simulink model "Mathematica_model"  (R2014a)
settings: Solver=ode5  SolverMode=SingleTasking  StartTime=0.0  StopTime=240  FixedStep=1e-6  RelTol=1e-3
InitFcn:
  | Mathematica_model_
values from neighbouring files (symbols this model uses):
  alpha = [alfa 0]    [Mathematica_model_.m]
  Cf = 1000e-6    (= 0.001)    [Mathematica_model_.m]
  CT1 = [34.2 88.9 129.8 148.6 139.3 123.3 69.9 25.5 15.1 10.5]    [Mathematica_model_.m]
  CT2 = [754.4 643.3 977.4 708.0 1119.7 970.2 733.8 708.0 359.8 170.7]    [Mathematica_model_.m]
  distance = [0 1 2 3 4 5 6 7 8 9 10 11 ... (2132 elements, 1x2132)]    [Track_data.mat]
  h_Mem = 5    [Mathematica_model_.m]
  h_Psi_s = 0.01    [Mathematica_model_.m]
  J = 0.043    [Mathematica_model_.m]
  Ki = Kp/Ti    (= 2.8)    [Mathematica_model_.m]
  Kp = 7    [Mathematica_model_.m]
  Kt = Ki/2    (= 1.4)    [Mathematica_model_.m]
  Lf = 1e-6    (= 1e-06)    [Mathematica_model_.m]
  Lm = 249.304e-3    (= 0.249304)    [Mathematica_model_.m]
  Lr = Lm+Llr    (= 0.255875)    [Mathematica_model_.m]
  Ls = Lm+Lls    (= 0.257335)    [Mathematica_model_.m]
  MInv = inv(M)    [Mathematica_model_.m]
  n_paralel = 10    [Mathematica_model_.m]
  n_serial = 162    [Mathematica_model_.m]
  pp = 2    [Mathematica_model_.m]
  Psi_rd_0 = Psi_dq_0(3)    [Mathematica_model_.m]
  Psi_sd_0 = Psi_dq_0(1)    [Mathematica_model_.m]
  Psi_sq_0 = Psi_dq_0(2)    [Mathematica_model_.m]
  Q0 = 4.8*3600    (= 17280)    [Mathematica_model_.m]
  R0 = [73 65 74 83 68 65 65 61 76 87].*1e-4    [Mathematica_model_.m]
  reduction = 2    [Mathematica_model_.m]
  Rf = 2000    [Mathematica_model_.m]
  Rs = 0.847    [Mathematica_model_.m]
  RT1 = [9.76 15 11 5.83 11 11 16 44 53 102].*1e-4    [Mathematica_model_.m]
  RT2 = [24 20 16 22 13 16 22 22 47 153].*1e-4    [Mathematica_model_.m]
  sigma = 1-Lm^2/(Lr*Ls)    (= 0.0560874089476)    [Mathematica_model_.m]
  SoC = [1 0.884 0.769 0.653 0.537 0.421 0.306 0.190 0.074 0]    [Mathematica_model_.m]
  speed = speedOptim    [Mathematica_model_.m]
  tauR = Lr/Rr    (= 0.384890192539)    [Mathematica_model_.m]
  Ts = 25e-6    (= 2.5e-05)    [Mathematica_model_.m]
  Tss = 500e-6    (= 0.0005)    [Mathematica_model_.m]
  Uoc = [4.19 4.06 3.93 3.86 3.8 3.76 3.72 3.6 3.43 3.05]    [Mathematica_model_.m]
  vehicle =     [Track_data.mat]
undefined symbols (not defined in the file or in its folder): DiscIntNeverNeededParam, Voltage
libraries: simulink x3
settings Model: SimulationMode=accelerator  NumberOfSteps=5  Creator=Jan  LastModifiedBy=Jan
settings DataIOCC: SignalLogging=off  DSMLogging=off
settings OptimizationCC: EfficientMapNaN2IntZero=off
settings DebuggingCC: MergeDetectMultiDrivingBlocksExec=error
settings HardwareCC: TargetLongLongMode=on  TargetIntDivRoundTo=Zero  TargetEndianess=LittleEndian  TargetHWDeviceType=MATLAB Host  ProdEqTarget=off
settings CodeAppCC: MaxIdLength=128
settings GRTTargetCC: CombineOutputUpdateFcns=off  GRTInterface=on

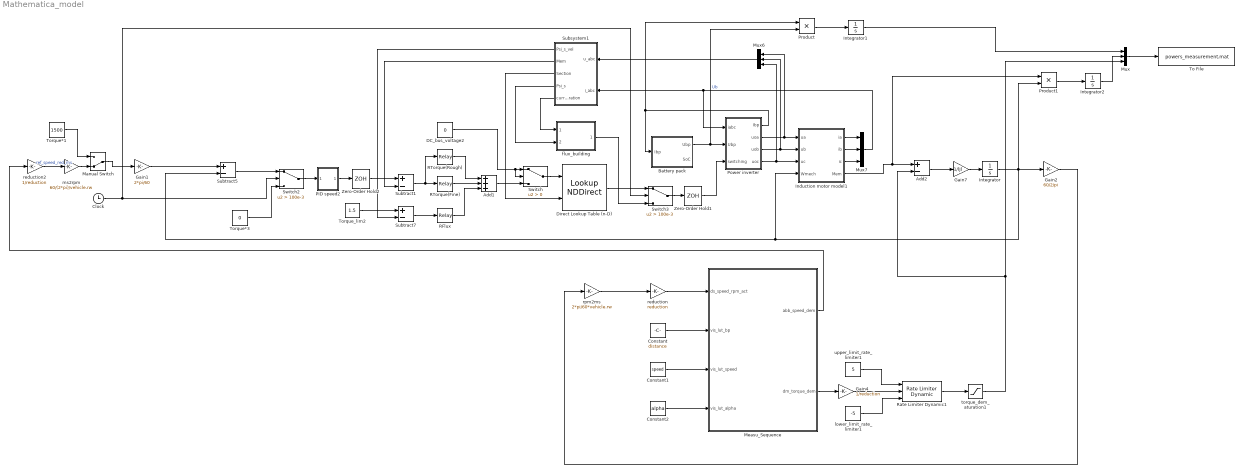
== system Mathematica_model ==
  Add1 : Sum  Inputs=+++
  Add2 : Sum  Inputs=+-
  Battery pack : Subsystem
  Clock : Clock
  Constant : Constant  Value=distance
  Constant1 : Constant  Value=speed
  Constant2 : Constant  Value=alpha
  DC_bus_voltage2 : Constant  Value=0
  Direct Lookup Table (n-D) : LookupNDDirect  NumberOfTableDimensions=3  InputsSelectThisObjectFromTable=Column  Table=Voltage  SampleTime=Ts
  Gain1 : Gain  Gain=2*pi/60
  Gain2 : Gain  Gain=60/2/pi
  Gain4 : Gain  Gain=1/reduction
  Gain7 : Gain  Gain=1/(J)
  Induction motor model1 : Subsystem
  Integrator : Integrator
  Integrator1 : Integrator
  Integrator2 : Integrator
  Manual Switch : ManualSwitch  CurrentSetting=0
  Measu_Sequence : Subsystem  TreatAsAtomicUnit=on
  Mux : Mux  Inputs=3
  Mux6 : Mux  Inputs=3
  Mux7 : Mux  Inputs=3
  PID speed2 : Subsystem
  Power inverter : Subsystem
  Product : Product
  Product1 : Product
  RFlux : Relay  OnSwitchValue=h_Psi_s  OffSwitchValue=-h_Psi_s
  RTorque(Fine) : Relay  OnSwitchValue=h_Mem  OffSwitchValue=-h_Mem  OnOutputValue=2
  RTorque(Rough) : Relay  OnSwitchValue=-h_Mem  OffSwitchValue=-2*h_Mem  OnOutputValue=0  OffOutputValue=4
  Rate Limiter Dynamic1 : simulink/Discontinuities/Rate Limiter Dynamic
  Subsystem1 : Subsystem
  Subtract1 : Sum  Inputs=+-
  Subtract5 : Sum  Inputs=+-
  Subtract7 : Sum  Inputs=+-
  Switch : Switch  Criteria=u2 > Threshold
  Switch2 : Switch  Criteria=u2 > Threshold  Threshold=100e-3
  Switch3 : Switch  Criteria=u2 > Threshold  Threshold=100e-3
  To File : ToFile  Filename=powers_measurement.mat  MatrixName=ans_2  SaveFormat=Timeseries  SampleTime=0.1
  Torque*1 : Constant  Value=1500
  Torque*3 : Constant  Value=0
  Torque_lim2 : Constant  Value=1.5
  Zero-Order Hold1 : ZeroOrderHold  SampleTime=50e-6
  Zero-Order Hold2 : ZeroOrderHold  SampleTime=Tss
  flux_building : Subsystem
  lower_limit_rate_limiter1 : Constant  Value=-5
  ms2rpm : Gain  Gain=60/(2*pi)/vehicle.rw
  reduction : Gain  Gain=reduction
  reduction2 : Gain  Gain=1/reduction
  rpm2ms : Gain  Gain=2*pi/60*vehicle.rw
  torque_dem_aturation1 : Saturate  UpperLimit=90  LowerLimit=-90  OutDataTypeStr=double
  upper_limit_rate_limiter1 : Constant  Value=5
  wires:
  Subsystem1/1(Psi_s_vel) -> Subtract7/2
  Power inverter/3(uob) -> Mux6/2, Induction motor model1/2(ub)
  Add2/1 -> Gain7/1
  Gain7/1 -> Integrator/1
  Induction motor model1/4(Mem) -> Product1/1, Add2/1
  Induction motor model1/2(ib) -> Mux7/2
  RFlux/1 -> Add1/3
  RTorque(Fine)/1 -> Add1/2
  RTorque(Rough)/1 -> Add1/1
  Add1/1 -> Switch/3
  Subtract7/1 -> RFlux/1
  Manual Switch/1 -> Gain1/1
  Induction motor model1/1(ia) -> Mux7/1
  Mux6/1 -> Subsystem1/1(u_abc)
  Power inverter/2(uoa) -> Induction motor model1/1(ua), Mux6/1
  Induction motor model1/3(ic) -> Mux7/3
  Power inverter/4(uoc) -> Mux6/3, Induction motor model1/3(uc)
  Mux7/1 -> Power inverter/1(iabc), Subsystem1/2(i_abc)
  Subsystem1/3(Section) -> Direct Lookup Table (n-D)/2
  DC_bus_voltage2/1 -> Switch/2, Switch/1
  Torque_lim2/1 -> Subtract7/1
  Switch/1 -> Direct Lookup Table (n-D)/1
  Subtract1/1 -> RTorque(Rough)/1, RTorque(Fine)/1
  Gain1/1 -> Subtract5/1
  PID speed2/1(y(t)) -> Zero-Order Hold2/1
  Subsystem1/4(Psi_s) -> flux_building/2(stator_flux)
  Subsystem1/5(curr_saturation) -> flux_building/1(current_sat)
  flux_building/1(voltage_vec) -> Switch3/3
  Subtract5/1 -> Switch2/1
  Torque*3/1 -> Switch2/3
  Direct Lookup Table (n-D)/1 -> Switch3/1
  Zero-Order Hold1/1 -> Power inverter/3(switching)
  Subsystem1/2(Mem) -> Subtract1/2
  Zero-Order Hold2/1 -> Subtract1/1
  Switch3/1 -> Zero-Order Hold1/1
  Switch2/1 -> PID speed2/1(e(t))
  Clock/1 -> Switch3/2, Switch2/2
  Measu_Sequence/2(dm_torque_dem) -> Gain4/1
  reduction/1 -> Measu_Sequence/1(ds_speed_rpm_act)
  rpm2ms/1 -> reduction/1
  reduction2/1 -> ms2rpm/1  "ref_speed_red_ms"
  Measu_Sequence/1(abb_speed_dem) -> reduction2/1
  Rate Limiter Dynamic1/1 -> torque_dem_aturation1/1
  lower_limit_rate_limiter1/1 -> Rate Limiter Dynamic1/3
  upper_limit_rate_limiter1/1 -> Rate Limiter Dynamic1/1
  Gain4/1 -> Rate Limiter Dynamic1/2
  Constant/1 -> Measu_Sequence/2(vis_lut_bp)
  Constant1/1 -> Measu_Sequence/3(vis_lut_speed)
  Constant2/1 -> Measu_Sequence/4(vis_lut_alpha)
  Product/1 -> Integrator1/1
  Product1/1 -> Integrator2/1
  ms2rpm/1 -> Manual Switch/2
  Integrator/1 -> Product1/2, Subtract5/2, Induction motor model1/4(Wmech), Gain2/1
  Gain2/1 -> rpm2ms/1
  Power inverter/1(Ibp) -> Product/1, Battery pack/1(Ibp)
  Mux/1 -> To File/1
  Integrator2/1 -> Mux/2
  Integrator1/1 -> Mux/1
  torque_dem_aturation1/1 -> Mux/3, Add2/2
  Torque*1/1 -> Manual Switch/1
  Battery pack/1(Ubp) -> Product/2, Power inverter/2(Ubp)  "Ub"

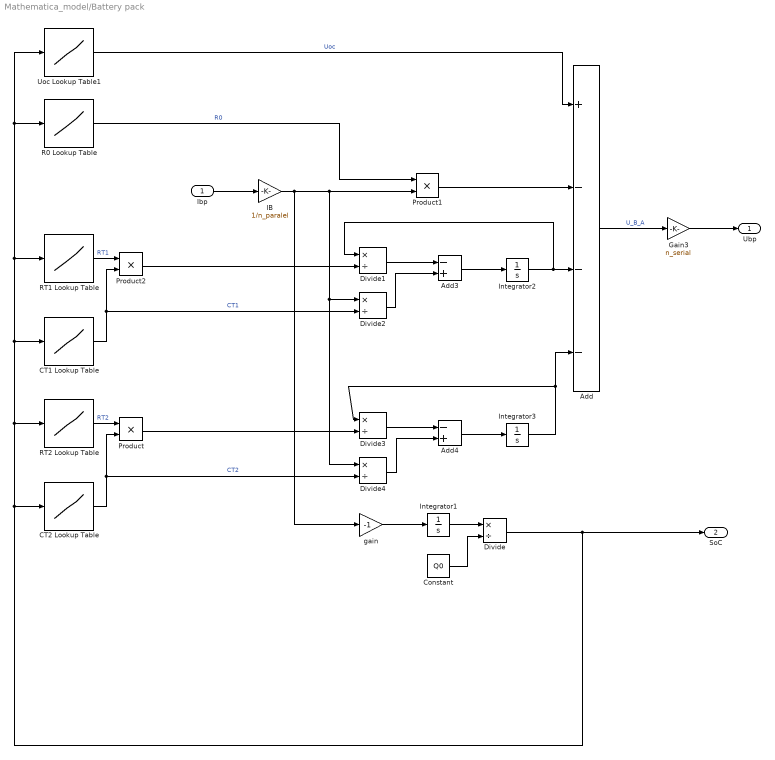
== system Mathematica_model/Battery pack ==
  Ibp : Inport
  Add : Sum  Inputs=+---
  Add3 : Sum  Inputs=-+
  Add4 : Sum  Inputs=-+
  CT1 Lookup Table : Lookup_n-D  NumberOfTableDimensions=1  BreakpointsForDimension1=SoC(10:-1:1)  Table=CT1(10:-1:1)  InternalRulePriority=Speed  RndMeth=Simplest  InputSameDT=on
  CT2 Lookup Table : Lookup_n-D  NumberOfTableDimensions=1  BreakpointsForDimension1=SoC(10:-1:1)  Table=CT2(10:-1:1)  InternalRulePriority=Speed  RndMeth=Simplest  InputSameDT=on
  Constant : Constant  Value=Q0
  Divide{,1..4} (5 alike) : Product  Inputs=*/
  Gain3 : Gain  Gain=n_serial
  IB : Gain  Gain=1/n_paralel
  Integrator1 : Integrator  InitialCondition=Q0
  Integrator2 : Integrator
  Integrator3 : Integrator
  Product : Product
  Product1 : Product
  Product2 : Product
  R0 Lookup Table : Lookup_n-D  NumberOfTableDimensions=1  BreakpointsForDimension1=SoC(10:-1:1)  Table=R0(10:-1:1)  InternalRulePriority=Speed  RndMeth=Simplest  InputSameDT=on
  RT1 Lookup Table : Lookup_n-D  NumberOfTableDimensions=1  BreakpointsForDimension1=SoC(10:-1:1)  Table=RT1(10:-1:1)  InternalRulePriority=Speed  RndMeth=Simplest  InputSameDT=on
  RT2 Lookup Table : Lookup_n-D  NumberOfTableDimensions=1  BreakpointsForDimension1=SoC(10:-1:1)  Table=RT2(10:-1:1)  InternalRulePriority=Speed  RndMeth=Simplest  InputSameDT=on
  Uoc Lookup Table1 : Lookup_n-D  NumberOfTableDimensions=1  BreakpointsForDimension1=SoC(10:-1:1)  Table=Uoc(10:-1:1)  InternalRulePriority=Speed  RndMeth=Simplest  InputSameDT=on
  gain : Gain  Gain=-1
  Ubp : Outport
  SoC : Outport  Port=2
  wires:
  Divide3/1 -> Add4/1
  Product1/1 -> Add/2
  Divide1/1 -> Add3/1
  Integrator3/1 -> Divide3/1, Add/4
  Divide4/1 -> Add4/2
  IB/1 -> gain/1, Divide2/1, Divide4/1, Product1/2
  Add4/1 -> Integrator3/1
  Divide2/1 -> Add3/2
  Add3/1 -> Integrator2/1
  Integrator2/1 -> Divide1/1, Add/3
  Add/1 -> Gain3/1  "U_B_A"
  Gain3/1 -> Ubp/1
  Ibp/1 -> IB/1
  gain/1 -> Integrator1/1
  Integrator1/1 -> Divide/1
  Constant/1 -> Divide/2
  Divide/1 -> RT1 Lookup Table/1, R0 Lookup Table/1, Uoc Lookup Table1/1, CT1 Lookup Table/1, RT2 Lookup Table/1, CT2 Lookup Table/1, SoC/1
  R0 Lookup Table/1 -> Product1/1  "R0"
  RT2 Lookup Table/1 -> Product/1  "RT2"
  CT2 Lookup Table/1 -> Product/2, Divide4/2  "CT2"
  RT1 Lookup Table/1 -> Product2/1  "RT1"
  CT1 Lookup Table/1 -> Divide2/2, Product2/2  "CT1"
  Uoc Lookup Table1/1 -> Add/1  "Uoc"
  Product2/1 -> Divide1/2
  Product/1 -> Divide3/2

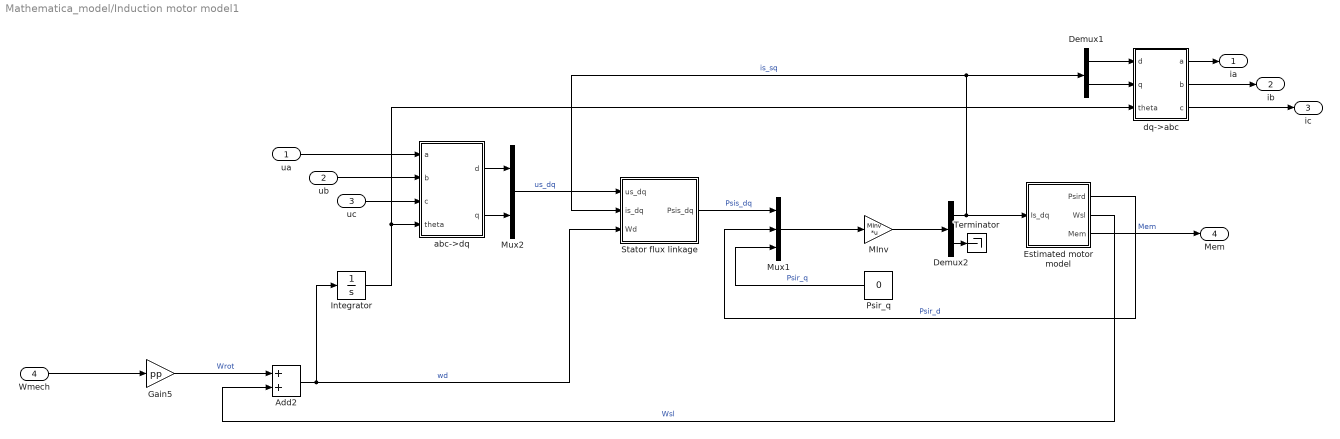
== system Mathematica_model/Induction motor model1 ==
  ua : Inport
  ub : Inport  Port=2
  uc : Inport  Port=3
  Wmech : Inport  Port=4
  Add2 : Sum
  Demux1 : Demux  Outputs=2
  Demux2 : Demux  Outputs=2
  Estimated motor model : Subsystem
  Gain5 : Gain  Gain=pp
  Integrator : Integrator
  MInv : Gain  Gain=MInv  Multiplication=Matrix(K*u)
  Mux1 : Mux  Inputs=3
  Mux2 : Mux  Inputs=2
  Psir_q : Constant  Value=0  VectorParams1D=off
  Stator flux linkage : Subsystem
  Terminator : Terminator
  abc->dq : Subsystem
  dq->abc : Subsystem
  ia : Outport
  ib : Outport  Port=2
  ic : Outport  Port=3
  Mem : Outport  Port=4
  wires:
  Add2/1 -> Integrator/1, Stator flux linkage/3(Wd)  "wd"
  Demux2/2 -> Terminator/1
  Mux2/1 -> Stator flux linkage/1(us_dq)  "us_dq"
  abc->dq/2(q) -> Mux2/2
  uc/1 -> abc->dq/3(c)
  ua/1 -> abc->dq/1(a)
  abc->dq/1(d) -> Mux2/1
  Stator flux linkage/1(Psis_dq) -> Mux1/1  "Psis_dq"
  ub/1 -> abc->dq/2(b)
  Mux1/1 -> MInv/1
  MInv/1 -> Demux2/1
  Psir_q/1 -> Mux1/3  "Psir_q"
  Demux2/1 -> Estimated motor model/1(Is_dq), Stator flux linkage/2(is_dq), Demux1/1  "is_sq"
  Estimated motor model/1(Psird) -> Mux1/2  "Psir_d"
  Estimated motor model/2(Wsl) -> Add2/2  "Wsl"
  Estimated motor model/3(Mem) -> Mem/1  "Mem"
  Demux1/1 -> dq->abc/1(d)
  Demux1/2 -> dq->abc/2(q)
  dq->abc/1(a) -> ia/1
  dq->abc/2(b) -> ib/1
  dq->abc/3(c) -> ic/1
  Integrator/1 -> dq->abc/3(theta), abc->dq/4(theta)
  Wmech/1 -> Gain5/1
  Gain5/1 -> Add2/1  "Wrot"

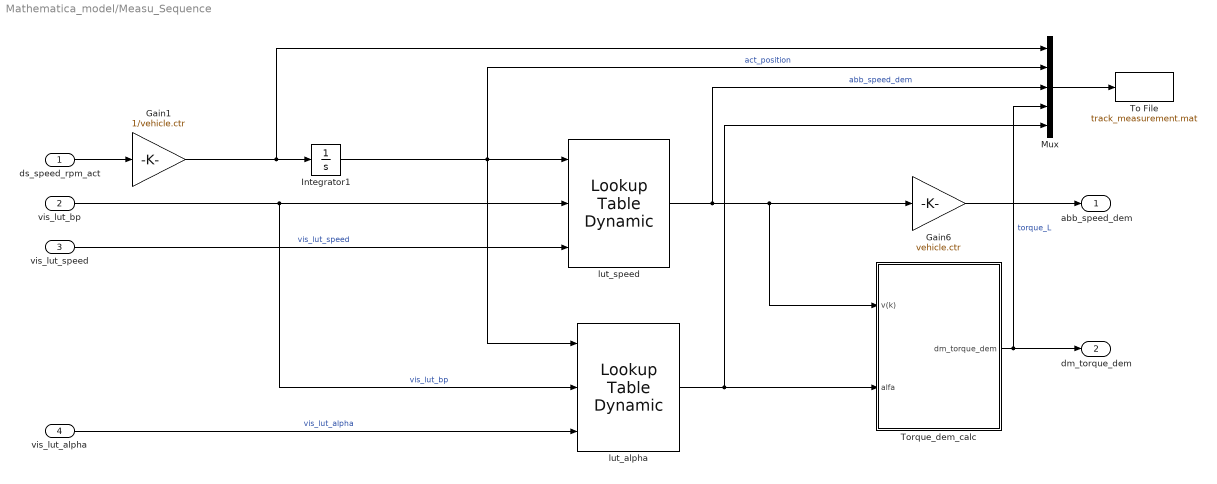
== system Mathematica_model/Measu_Sequence ==
  ds_speed_rpm_act : Inport
  vis_lut_bp : Inport  Port=2
  vis_lut_speed : Inport  Port=3
  vis_lut_alpha : Inport  Port=4
  Gain1 : Gain  Gain=1/vehicle.ctr
  Gain6 : Gain  Gain=vehicle.ctr
  Integrator1 : Integrator
  Mux : Mux  Inputs=5
  To File : ToFile  Filename=track_measurement.mat  SaveFormat=Timeseries  SampleTime=0.1
  Torque_dem_calc : Subsystem
  lut_alpha : simulink/Lookup Tables/Lookup Table Dynamic  LookUpMeth=Interpolation-Use End Values  OutDataTypeStr=fixdt('double')  OutputDataTypeScalingMode=Specify via dialog  OutDataType=fixdt('double')  OutScaling=2^-10  DoSatur=off
  lut_speed : simulink/Lookup Tables/Lookup Table Dynamic  LookUpMeth=Interpolation-Use End Values  OutDataTypeStr=fixdt('double')  OutputDataTypeScalingMode=Specify via dialog  OutDataType=fixdt('double')  OutScaling=2^-10  DoSatur=off
  abb_speed_dem : Outport
  dm_torque_dem : Outport  Port=2
  wires:
  Integrator1/1 -> lut_alpha/1, Mux/2, lut_speed/1  "act_position"
  Torque_dem_calc/1(dm_torque_dem) -> Mux/4, dm_torque_dem/1  "torque_L"
  vis_lut_bp/1 -> lut_alpha/2, lut_speed/2  "vis_lut_bp"
  vis_lut_speed/1 -> lut_speed/3  "vis_lut_speed"
  vis_lut_alpha/1 -> lut_alpha/3  "vis_lut_alpha"
  Gain6/1 -> abb_speed_dem/1
  lut_speed/1 -> Mux/3, Torque_dem_calc/1(v(k)), Gain6/1  "abb_speed_dem"
  lut_alpha/1 -> Mux/5, Torque_dem_calc/2(alfa)
  ds_speed_rpm_act/1 -> Gain1/1
  Gain1/1 -> Mux/1, Integrator1/1
  Mux/1 -> To File/1

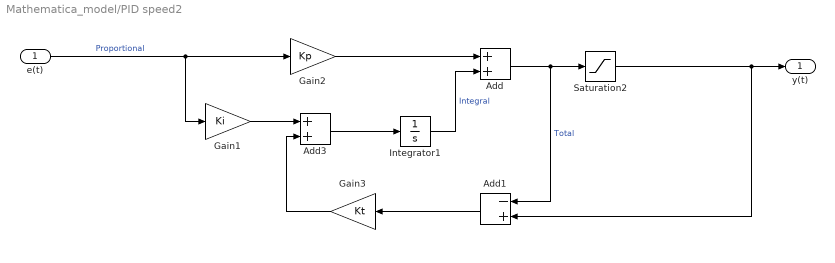
== system Mathematica_model/PID speed2 ==
  e(t) : Inport
  Add : Sum
  Add1 : Sum  Inputs=-+
  Add3 : Sum
  Gain1 : Gain  Gain=Ki
  Gain2 : Gain  Gain=Kp
  Gain3 : Gain  Gain=Kt
  Integrator1 : Integrator
  Saturation2 : Saturate  UpperLimit=70*2  LowerLimit=-70*1
  y(t) : Outport
  wires:
  e(t)/1 -> Gain2/1, Gain1/1  "Proportional"
  Add3/1 -> Integrator1/1
  Gain1/1 -> Add3/1
  Add/1 -> Saturation2/1, Add1/1  "Total"
  Add1/1 -> Gain3/1
  Integrator1/1 -> Add/2  "Integral"
  Gain2/1 -> Add/1
  Gain3/1 -> Add3/2
  Saturation2/1 -> Add1/2, y(t)/1

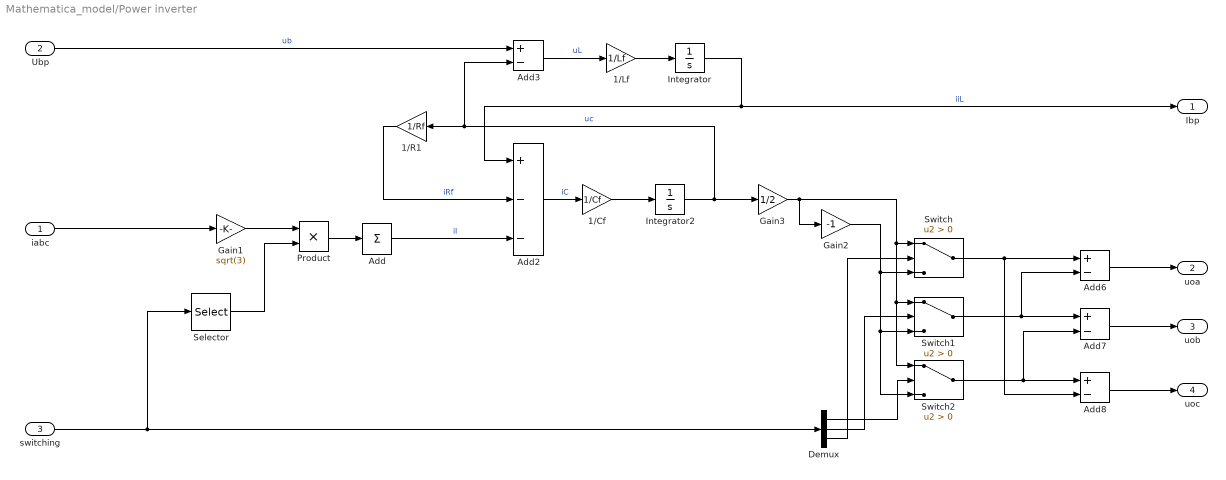
== system Mathematica_model/Power inverter ==
  iabc : Inport
  Ubp : Inport  Port=2
  switching : Inport  Port=3
  1/Cf : Gain  Gain=1/Cf
  1/Lf : Gain  Gain=1/Lf
  1/R1 : Gain  Gain=1/Rf
  Add : Sum  Inputs=+
  Add2 : Sum  Inputs=+--
  Add{3,6..8} (4 alike) : Sum  Inputs=+-
  Demux : Demux  Outputs=3
  Gain1 : Gain  Gain=sqrt(3)
  Gain2 : Gain  Gain=-1
  Gain3 : Gain  Gain=1/2
  Integrator : Integrator
  Integrator2 : Integrator  InitialCondition=560
  Product : Product
  Selector : Selector  InputPortWidth=3  Indices=[3 2 1]
  Switch : Switch  Criteria=u2 > Threshold  SampleTime=Ts
  Switch1 : Switch  Criteria=u2 > Threshold  SampleTime=Ts
  Switch2 : Switch  Criteria=u2 > Threshold  SampleTime=Ts
  Ibp : Outport
  uoa : Outport  Port=2
  uob : Outport  Port=3
  uoc : Outport  Port=4
  wires:
  Switch/1 -> Add8/2, Add6/1
  Switch1/1 -> Add6/2, Add7/1
  Switch2/1 -> Add7/2, Add8/1
  Gain2/1 -> Switch2/3, Switch1/3, Switch/3
  Add8/1 -> uoc/1
  Add7/1 -> uob/1
  Add6/1 -> uoa/1
  Demux/2 -> Switch1/2
  Demux/3 -> Switch/2
  Demux/1 -> Switch2/2
  iabc/1 -> Gain1/1
  Selector/1 -> Product/2
  Product/1 -> Add/1
  switching/1 -> Demux/1, Selector/1
  1/Lf/1 -> Integrator/1
  Add3/1 -> 1/Lf/1  "uL"
  1/Cf/1 -> Integrator2/1
  Add2/1 -> 1/Cf/1  "iC"
  Add/1 -> Add2/3  "iI"
  1/R1/1 -> Add2/2  "iRf"
  Integrator2/1 -> Add3/2, 1/R1/1, Gain3/1  "uc"
  Integrator/1 -> Add2/1, Ibp/1  "iiL"
  Ubp/1 -> Add3/1  "ub"
  Gain3/1 -> Gain2/1, Switch/1, Switch2/1, Switch1/1
  Gain1/1 -> Product/1

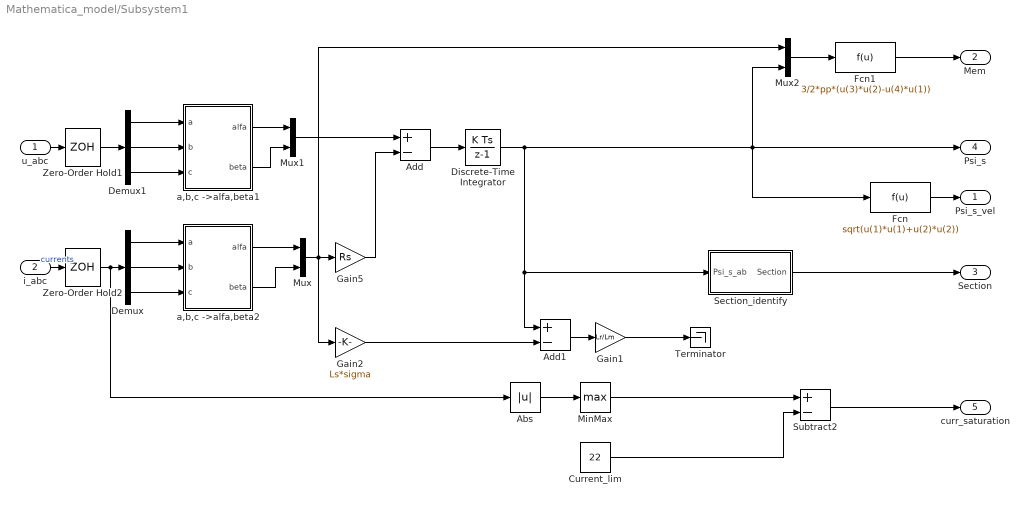
== system Mathematica_model/Subsystem1 ==
  u_abc : Inport
  i_abc : Inport  Port=2
  Abs : Abs
  Add : Sum  Inputs=+-
  Add1 : Sum  Inputs=+-
  Current_lim : Constant  Value=22
  Demux : Demux  Outputs=3
  Demux1 : Demux  Outputs=3
  Discrete-Time Integrator : DiscreteIntegrator  InitialConditionSetting=State (most efficient)  SampleTime=Ts  ICPrevOutput=DiscIntNeverNeededParam  ICPrevScaledInput=DiscIntNeverNeededParam
  Fcn : Fcn  Expr=sqrt(u(1)*u(1)+u(2)*u(2))
  Fcn1 : Fcn  Expr=3/2*pp*(u(3)*u(2)-u(4)*u(1))
  Gain1 : Gain  Gain=Lr/Lm
  Gain2 : Gain  Gain=Ls*sigma
  Gain5 : Gain  Gain=Rs
  MinMax : MinMax  Function=max
  Mux : Mux  Inputs=2
  Mux1 : Mux  Inputs=2
  Mux2 : Mux  Inputs=2
  Section_identify : Subsystem
  Subtract2 : Sum  Inputs=+-
  Terminator : Terminator
  Zero-Order Hold1 : ZeroOrderHold  SampleTime=Ts
  Zero-Order Hold2 : ZeroOrderHold  SampleTime=Ts
  a,b,c ->alfa,beta1 : Subsystem
  a,b,c ->alfa,beta2 : Subsystem
  Psi_s_vel : Outport
  Mem : Outport  Port=2
  Section : Outport  Port=3
  Psi_s : Outport  Port=4
  curr_saturation : Outport  Port=5
  wires:
  a,b,c ->alfa,beta2/1(alfa) -> Mux/1
  a,b,c ->alfa,beta2/2(beta) -> Mux/2
  a,b,c ->alfa,beta1/1(alfa) -> Mux1/1
  a,b,c ->alfa,beta1/2(beta) -> Mux1/2
  Demux/1 -> a,b,c ->alfa,beta2/1(a)
  Demux/3 -> a,b,c ->alfa,beta2/3(c)
  Demux/2 -> a,b,c ->alfa,beta2/2(b)
  Demux1/1 -> a,b,c ->alfa,beta1/1(a)
  Demux1/2 -> a,b,c ->alfa,beta1/2(b)
  Demux1/3 -> a,b,c ->alfa,beta1/3(c)
  Mux/1 -> Mux2/1, Gain2/1, Gain5/1
  Mux1/1 -> Add/1
  Gain5/1 -> Add/2
  Add/1 -> Discrete-Time Integrator/1
  Add1/1 -> Gain1/1
  Gain2/1 -> Add1/2
  Gain1/1 -> Terminator/1
  u_abc/1 -> Zero-Order Hold1/1
  Zero-Order Hold1/1 -> Demux1/1
  Zero-Order Hold2/1 -> Abs/1, Demux/1
  Discrete-Time Integrator/1 -> Psi_s/1, Fcn/1, Mux2/2, Add1/1, Section_identify/1(Psi_s_ab)
  Fcn/1 -> Psi_s_vel/1
  Mux2/1 -> Fcn1/1
  Fcn1/1 -> Mem/1
  Section_identify/1(Section) -> Section/1
  i_abc/1 -> Zero-Order Hold2/1  "currents"
  MinMax/1 -> Subtract2/1
  Abs/1 -> MinMax/1
  Current_lim/1 -> Subtract2/2
  Subtract2/1 -> curr_saturation/1

== system Mathematica_model/flux_building ==
  current_sat : Inport
  stator_flux : Inport  Port=2
  Product : Product
  RFlux1 : Relay  OnSwitchValue=0.01  OffSwitchValue=-0.01  OnOutputValue=[0 0 0]  OffOutputValue=[1 1 1]
  RFlux2 : Relay  OnSwitchValue=0.001  OffSwitchValue=-0.001  OnOutputValue=[1 0 1]  OffOutputValue=[0 0 1]
  Selector : Selector  InputPortWidth=2  Indices=[2]
  voltage_vec : Outport
  wires:
  current_sat/1 -> RFlux1/1
  stator_flux/1 -> Selector/1
  Selector/1 -> RFlux2/1
  RFlux1/1 -> Product/1
  RFlux2/1 -> Product/2
  Product/1 -> voltage_vec/1

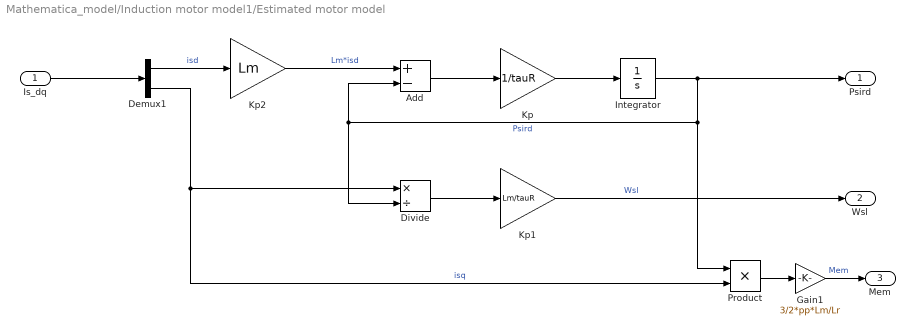
== system Mathematica_model/Induction motor model1/Estimated motor model ==
  Is_dq : Inport
  Add : Sum  Inputs=+-
  Demux1 : Demux  Outputs=2
  Divide : Product  Inputs=*/
  Gain1 : Gain  Gain=3/2*pp*Lm/Lr
  Integrator : Integrator  InitialCondition=Psi_rd_0
  Kp : Gain  Gain=1/tauR
  Kp1 : Gain  Gain=Lm/tauR
  Kp2 : Gain  Gain=Lm
  Product : Product
  Psird : Outport
  Wsl : Outport  Port=2
  Mem : Outport  Port=3
  wires:
  Is_dq/1 -> Demux1/1
  Demux1/1 -> Kp2/1  "isd"
  Kp2/1 -> Add/1  "Lm*isd"
  Add/1 -> Kp/1
  Kp/1 -> Integrator/1
  Integrator/1 -> Divide/2, Add/2, Product/1, Psird/1  "Psird"
  Demux1/2 -> Product/2, Divide/1  "isq"
  Divide/1 -> Kp1/1
  Kp1/1 -> Wsl/1  "Wsl"
  Product/1 -> Gain1/1
  Gain1/1 -> Mem/1  "Mem"

== system Mathematica_model/Induction motor model1/Stator flux linkage ==
  us_dq : Inport
  is_dq : Inport  Port=2
  Wd : Inport  Port=3
  Add3 : Sum  Inputs=+--
  Constant : Constant  Value=[0 -1;1 0]  VectorParams1D=off
  Gain : Gain  Gain=Rs
  Integrator : Integrator  InitialCondition=[Psi_sd_0 Psi_sq_0]
  Product : Product
  Product1 : Product  Multiplication=Matrix(*)
  Psis_dq : Outport
  wires:
  us_dq/1 -> Add3/1
  is_dq/1 -> Gain/1
  Gain/1 -> Add3/2
  Wd/1 -> Product/1
  Constant/1 -> Product/2
  Product/1 -> Product1/1
  Product1/1 -> Add3/3
  Add3/1 -> Integrator/1
  Integrator/1 -> Product1/2, Psis_dq/1

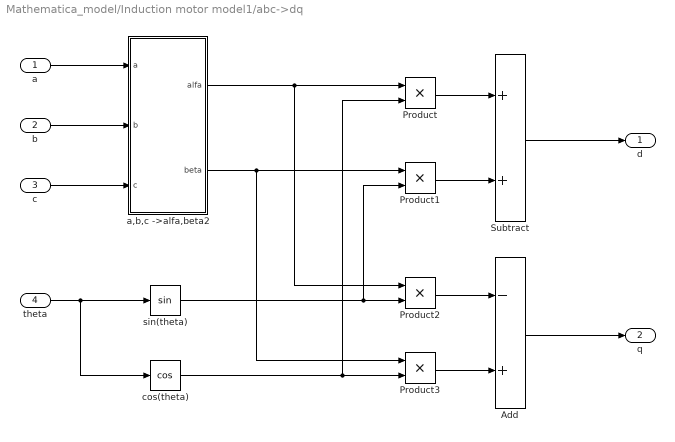
== system Mathematica_model/Induction motor model1/abc->dq ==
  a : Inport
  b : Inport  Port=2
  c : Inport  Port=3
  theta : Inport  Port=4
  Add : Sum  Inputs=-+
  Product{,1..3} (4 alike) : Product
  Subtract : Sum
  a,b,c ->alfa,beta2 : Subsystem
  cos(theta) : Trigonometry  Operator=cos
  sin(theta) : Trigonometry
  d : Outport
  q : Outport  Port=2
  wires:
  c/1 -> a,b,c ->alfa,beta2/3(c)
  b/1 -> a,b,c ->alfa,beta2/2(b)
  a/1 -> a,b,c ->alfa,beta2/1(a)
  Add/1 -> q/1
  Product3/1 -> Add/2
  Product2/1 -> Add/1
  Subtract/1 -> d/1
  Product1/1 -> Subtract/2
  Product/1 -> Subtract/1
  sin(theta)/1 -> Product1/2, Product2/2
  a,b,c ->alfa,beta2/2(beta) -> Product3/1, Product1/1
  cos(theta)/1 -> Product/2, Product3/2
  a,b,c ->alfa,beta2/1(alfa) -> Product/1, Product2/1
  theta/1 -> sin(theta)/1, cos(theta)/1

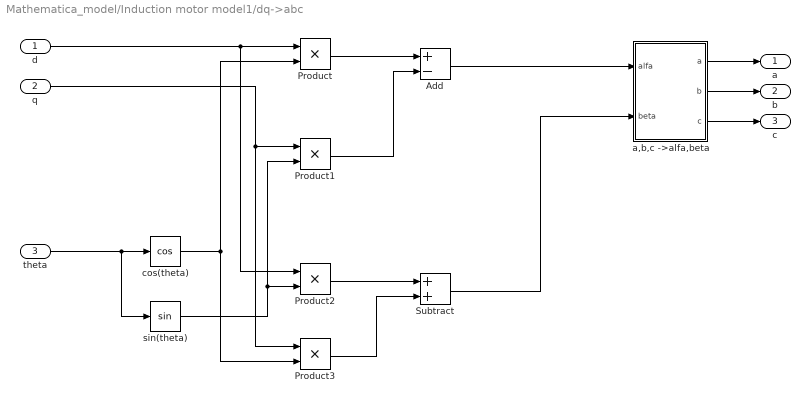
== system Mathematica_model/Induction motor model1/dq->abc ==
  d : Inport
  q : Inport  Port=2
  theta : Inport  Port=3
  Add : Sum  Inputs=+-
  Product{,1..3} (4 alike) : Product
  Subtract : Sum
  a,b,c ->alfa,beta : Subsystem
  cos(theta) : Trigonometry  Operator=cos
  sin(theta) : Trigonometry
  a : Outport
  b : Outport  Port=2
  c : Outport  Port=3
  wires:
  Subtract/1 -> a,b,c ->alfa,beta/2(beta)
  q/1 -> Product1/1, Product3/1
  Add/1 -> a,b,c ->alfa,beta/1(alfa)
  d/1 -> Product/1, Product2/1
  a,b,c ->alfa,beta/3(c) -> c/1
  a,b,c ->alfa,beta/2(b) -> b/1
  a,b,c ->alfa,beta/1(a) -> a/1
  cos(theta)/1 -> Product3/2, Product/2
  theta/1 -> sin(theta)/1, cos(theta)/1
  Product/1 -> Add/1
  sin(theta)/1 -> Product1/2, Product2/2
  Product1/1 -> Add/2
  Product2/1 -> Subtract/1
  Product3/1 -> Subtract/2

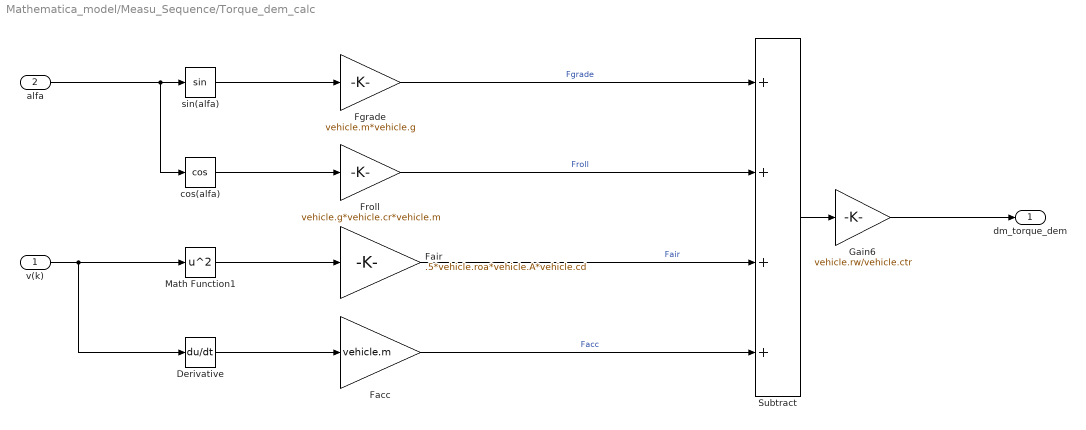
== system Mathematica_model/Measu_Sequence/Torque_dem_calc ==
  v(k) : Inport
  alfa : Inport  Port=2
  Derivative : Derivative
  Facc : Gain  Gain=vehicle.m
  Fair : Gain  Gain=.5*vehicle.roa*vehicle.A*vehicle.cd
  Fgrade : Gain  Gain=vehicle.m*vehicle.g
  Froll : Gain  Gain=vehicle.g*vehicle.cr*vehicle.m
  Gain6 : Gain  Gain=vehicle.rw/vehicle.ctr
  Math Function1 : Math  Operator=square  SaturateOnIntegerOverflow=on
  Subtract : Sum  Inputs=++++
  cos(alfa) : Trigonometry  Operator=cos
  sin(alfa) : Trigonometry
  dm_torque_dem : Outport
  wires:
  Subtract/1 -> Gain6/1
  Froll/1 -> Subtract/2  "Froll"
  alfa/1 -> cos(alfa)/1, sin(alfa)/1
  sin(alfa)/1 -> Fgrade/1
  cos(alfa)/1 -> Froll/1
  Fgrade/1 -> Subtract/1  "Fgrade"
  Fair/1 -> Subtract/3  "Fair"
  Math Function1/1 -> Fair/1
  Facc/1 -> Subtract/4  "Facc"
  Gain6/1 -> dm_torque_dem/1
  v(k)/1 -> Derivative/1, Math Function1/1
  Derivative/1 -> Facc/1

== system Mathematica_model/Subsystem1/Section_identify ==
  Psi_s_ab : Inport
  1-D Lookup Table : Lookup_n-D  NumberOfTableDimensions=1  BreakpointsForDimension1=[0;2*pi/6;4*pi/6;6*pi/6;8*pi/6;10*pi/6;2*pi]  Table=[0;1;2;3;4;5;0]  InterpMethod=Flat  InternalRulePriority=Speed  RndMeth=Simplest  InputSameDT=on
  Add3 : Sum
  Angel_offset1 : Constant  Value=2*pi
  Complex to Magnitude-Angle : ComplexToMagnitudeAngle
  Demux1 : Demux  Outputs=2
  Real-Imag to Complex : RealImagToComplex
  Switch : Switch  Criteria=u2 > Threshold
  Section : Outport
  wires:
  Angel_offset1/1 -> Add3/2
  Add3/1 -> Switch/3
  1-D Lookup Table/1 -> Section/1
  Real-Imag to Complex/1 -> Complex to Magnitude-Angle/1
  Demux1/2 -> Real-Imag to Complex/2
  Demux1/1 -> Real-Imag to Complex/1
  Psi_s_ab/1 -> Demux1/1
  Complex to Magnitude-Angle/2 -> Switch/1, Switch/2, Add3/1
  Switch/1 -> 1-D Lookup Table/1

== system Mathematica_model/Subsystem1/a,b,c ->alfa,beta1 ==
  a : Inport
  b : Inport  Port=2
  c : Inport  Port=3
  Gain3 : Gain  Gain=2*(3^.5)/3
  Gain4 : Gain  Gain=(3^.5/3)
  Subtract1 : Sum  Inputs=--
  Terminator : Terminator
  alfa : Outport
  beta : Outport  Port=2
  wires:
  a/1 -> Gain4/1, alfa/1
  c/1 -> Gain3/1
  Gain3/1 -> Subtract1/2
  Gain4/1 -> Subtract1/1
  Subtract1/1 -> beta/1
  b/1 -> Terminator/1

== system Mathematica_model/Subsystem1/a,b,c ->alfa,beta2 ==
  a : Inport
  b : Inport  Port=2
  c : Inport  Port=3
  Gain3 : Gain  Gain=2*(3^.5)/3
  Gain4 : Gain  Gain=(3^.5/3)
  Subtract1 : Sum  Inputs=--
  Terminator : Terminator
  alfa : Outport
  beta : Outport  Port=2
  wires:
  b/1 -> Terminator/1
  Subtract1/1 -> beta/1
  Gain4/1 -> Subtract1/1
  Gain3/1 -> Subtract1/2
  c/1 -> Gain3/1
  a/1 -> alfa/1, Gain4/1

== system Mathematica_model/Induction motor model1/abc->dq/a,b,c ->alfa,beta2 ==
  a : Inport
  b : Inport  Port=2
  c : Inport  Port=3
  Gain1 : Gain  Gain=2*sqrt(3)/3
  Gain2 : Gain  Gain=sqrt(3)/3
  Subtract1 : Sum
  Terminator : Terminator
  alfa : Outport
  beta : Outport  Port=2
  wires:
  a/1 -> Gain2/1, alfa/1
  Gain2/1 -> Subtract1/1
  c/1 -> Terminator/1
  b/1 -> Gain1/1
  Subtract1/1 -> beta/1
  Gain1/1 -> Subtract1/2

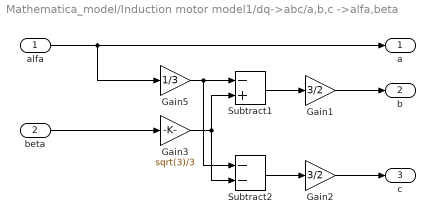
== system Mathematica_model/Induction motor model1/dq->abc/a,b,c ->alfa,beta ==
  alfa : Inport
  beta : Inport  Port=2
  Gain1 : Gain  Gain=3/2
  Gain2 : Gain  Gain=3/2
  Gain3 : Gain  Gain=sqrt(3)/3
  Gain5 : Gain  Gain=1/3
  Subtract1 : Sum  Inputs=-+
  Subtract2 : Sum  Inputs=--
  a : Outport
  b : Outport  Port=2
  c : Outport  Port=3
  wires:
  alfa/1 -> Gain5/1, a/1
  Gain5/1 -> Subtract2/1, Subtract1/1
  beta/1 -> Gain3/1
  Gain3/1 -> Subtract1/2, Subtract2/2
  Subtract2/1 -> Gain2/1
  Subtract1/1 -> Gain1/1
  Gain1/1 -> b/1
  Gain2/1 -> c/1
